simulink model "thrust2omega"  (Simulink 9.2)
settings: Solver=ode3  StartTime=0.0  StopTime=10.0  FixedStep=Ts  RelTol=1e-3  EnableMultiTasking=on
values from neighbouring files (symbols this model uses):
  b = 2e-09    [dataset.mat]    (also in initiateVars.m; system_workspace.mat; system_workspace_ayk.mat)
  k = 2.2e-08    [dataset.mat]    (also in initiateVars.m; system_workspace.mat; system_workspace_ayk.mat)
  l = 0.046    [dataset.mat]    (also in initiateVars.m; system_workspace.mat; system_workspace_ayk.mat)
settings Model: Creator=mgreiff  LastModifiedBy=aykut
settings DataIOCC: LimitDataPoints=off  SaveFormat=Dataset  SignalLoggingSaveFormat=Dataset
settings DebuggingCC: UnderspecifiedInitializationDetection=Simplified  MergeDetectMultiDrivingBlocksExec=error  FcnCallInpInsideContextMsg=error  StateNameClashWarn=none  SFExecutionAtInitializationDiag=warning
settings HardwareCC: ProdBitPerPointer=64  ProdBitPerSizeT=64  ProdBitPerPtrDiffT=64  ProdLargestAtomicFloat=Float  ProdIntDivRoundTo=Zero  ProdEndianess=LittleEndian  ProdWordSize=64  ProdHWDeviceType=Intel->x86-64 (Windows64)
settings ModelReferenceCC: PropagateSignalLabelsOutOfModel=on
settings GRTTargetCC: CombineOutputUpdateFcns=on  GRTInterface=off

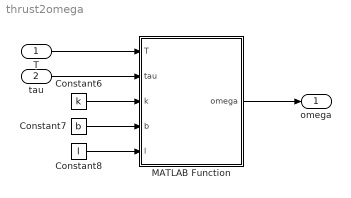
== system thrust2omega ==
  T : Inport  PortDimensions=1
  tau : Inport  Port=2  PortDimensions=3
  Constant6 : Constant  Value=k
  Constant7 : Constant  Value=b
  Constant8 : Constant  Value=l
  MATLAB Function : MATLAB Function  TreatAsAtomicUnit=on
  omega : Outport  PortDimensions=4
  wires:
  Constant7/1 -> MATLAB Function/4(b)
  tau/1 -> MATLAB Function/2(tau)
  Constant6/1 -> MATLAB Function/3(k)
  MATLAB Function/1(omega) -> omega/1
  T/1 -> MATLAB Function/1(T)
  Constant8/1 -> MATLAB Function/5(l)

== matlab function MATLAB Function ==
  data: T input double; omega output double; tau input double; k input double; b input double; l input double
function omega = Mw(T, tau, k, b, l)
%#codegen
tau_phi = tau(1);
tau_theta = tau(2);
tau_psi = tau(3);
w1sq = T/(4*k) - tau_theta/(2*k*l) - tau_psi / (4*b);
w2sq = T/(4*k) - tau_phi/(2*k*l) + tau_psi / (4*b);
w3sq = T/(4*k) + tau_theta/(2*k*l) - tau_psi / (4*b);
w4sq = T/(4*k) + tau_phi/(2*k*l) + tau_psi / (4*b);

omega = sqrt(max([w1sq w2sq w3sq w4sq]', 0));
